simulink model "SensorlessHeartBeatEstimate"  (R2017b)
settings: Solver=VariableStepAuto  StartTime=0.0  StopTime=120  RelTol=1e-3
libraries: slident x2, dspsigops x1
settings Model: Creator=prave  LastModifiedBy=prave

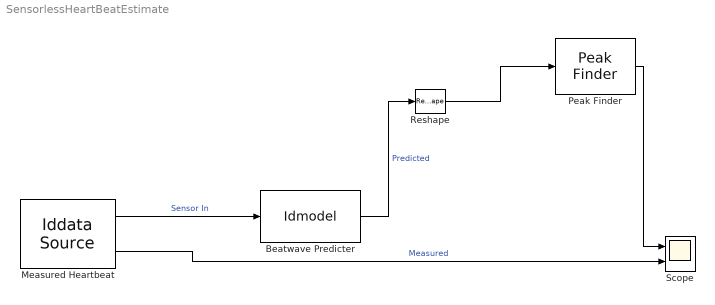
== system SensorlessHeartBeatEstimate ==
  Beatwave Predicter : slident/Models/Idmodel  sys=beat_mp  IC=x0  noi=on  seed=[]
      settings: SourceProductName=System Identification Toolbox  SourceProductBaseCode=ID
  Measured Heartbeat : slident/Iddata Source  iddataobj=beat
      settings: SourceProductName=System Identification Toolbox  SourceProductBaseCode=ID
  Peak Finder : dspsigops/Peak Finder  polarity=Maxima and Minima  outputIdx=off  outputVal=off  maxPeaks=10  NoiseDistinguish=off  thresh=0  roundingMode=Floor  overflowMode=off
      settings: SourceProductName=DSP System Toolbox  SourceProductBaseCode=DS  allowOverrides=off
  Reshape : Reshape
  Scope : Scope  NumInputPorts=2
  wires:
  Measured Heartbeat/1 -> Beatwave Predicter/1  "Sensor In"
  Beatwave Predicter/1 -> Reshape/1  "Predicted"
  Measured Heartbeat/2 -> Scope/2  "Measured"
  Peak Finder/1 -> Scope/1
  Reshape/1 -> Peak Finder/1
